simulink model "thermostat_model"  (R2024a)
settings: Solver=VariableStepAuto  StartTime=0.0  StopTime=10.0  RelTol=1e-3
StartFcn:
  | learning.simulink.modelCallbacks.startFunction(gcs)
StopFcn:
  | learning.simulink.modelCallbacks.stopFunction(gcs);
model workspace (MAT data in the model file):
  courseObject.course = 'simulink'
  courseObject.chapter = 12
  courseObject.lesson = 1
  courseObject.section = 3
  courseObject.task = 1
  t_ans = [0; 3.44882310802e-07; 2.06929386481e-06; 1.06913516349e-05; 5.38016404852e-05; 0.000269353084737; 0.00134711030599; 0.00673589641228; 0.0246147261548; 0.0493860964287; 0.083811385317; 0.129621810728; 0.15; 0.22645050849; 0.3; 0.398234685339; 0.45; 0.55; 0.6; 0.7; 0.75; 0.85; 0.9; 1; 1.05; 1.15; 1.2; 1.3; 1.35; 1.45; 1.5; 1.6; 1.65; 1.75; 1.8; 1.9; 1.95; 2.05; 2.1; 2.2; 2.25; 2.35; 2.4; 2.5; 2.55; 2.65; 2.7; 2.8; 2.85; 2.95; 3; 3.1; 3.15; 3.25; 3.3; 3.4; 3.45; 3.55; 3.6; 3.7; 3.75; 3.85; 3.9; 4; 4.05; 4.15; 4.2; 4.3; 4.35; 4.45; 4.5; 4.6; 4.65; 4.75; 4.8; 4.9; 4.95; 5.05; 5.1; 5.2; 5.25; 5.35; 5.4; 5.5; 5.55; 5.65; 5.7; 5.8; 5.85; 5.95; 6; 6.1; 6.15; 6.25; 6.3; 6.4; 6.45; 6.55; 6.6; 6.7; 6.75; 6.85; 6.9; 7; 7.05; 7.15; 7.2; 7.3; 7.35; 7.45; 7.5; 7.6; 7.65; 7.75; 7.8; 7.9; 7.95; 8.05; 8.1; 8.2; 8.25; 8.35; 8.4; 8.5; 8.55; 8.65; 8.7; 8.8; 8.85; 8.95; 9; 9.1; 9.15; 9.25; 9.3; 9.4; 9.45; 9.55; 9.6; 9.7; 9.75; 9.85; 9.9; 10]
  y_ans5 = [0.165; 0.164998492878; 0.164990957572; 0.164953288613; 0.164765132939; 0.163829066348; 0.159264513798; 0.139100169013; 0.2995349504; 0.280074861211; 0.411854808282; 0.399795884174; 0.507975423128; 0.592283569821; 0.667978066267; 0.737391490069; 0.802224756514; 0.863718172807; 0.922776170802; 0.980058262091; 1.03604536244; 1.09108815556; 1.14544235997; 1.19929444559; 1.25278038625; 1.30599933405; 1.35902359069; 1.41190587857; 1.46468464284; 1.51738791771; 1.57003614572; 1.62264423356; 1.6752230512; 1.72778052502; 1.78032243492; 1.83285299561; 1.88537528046; 1.93789153057; 1.99040338015; 2.04291202086; 2.09541832167; 2.14792291622; 2.20042626656; 2.25292870963; 2.30543049112; 2.35793179018; 2.41043273745; 2.4629334282; 2.5154339319; 2.56793429919; 2.62043456702; 2.67293476233; 2.72543490474; 2.77793500859; 2.83043508432; 2.88293513954; 2.9354351798; 2.98793520917; 3.04043523058; 3.09293524619]
  y_ans6 = [0; 0.000200949591965; 0.00120565787659; 0.00622820760954; 0.0313161877119; 0.156139821616; 0.765211136192; 3.47456129023; 9.66726186092; 14.4061638265; 17.7295717319; 19.7232109637; 20.7317148909; 20.8320685771; 21.5492269455; 21.892543187; 21.9704589902; 22.0381744411; 22.0479848156; 22.0487790728; 22.0492616288; 22.0494820492; 22.0494809578; 22.0492919817; 22.0489432093; 22.0484582994; 22.0478573326; 22.0471574743; 22.046373495; 22.045518183; 22.0446026738; 22.0436367161; 22.0426288871; 22.0415867683; 22.04051709; 22.0394258499; 22.0383184121; 22.0371995888; 22.0360737088; 22.0349446741; 22.0338160089; 22.0326908988; 22.0315722257; 22.030462596; 22.0293643652; 22.028279659; 22.0272103905; 22.0261582765; 22.0251248498; 22.024111472; 22.0231193432; 22.022149512; 22.0212028836; 22.0202802279; 22.0193821871; 22.0185092827; 22.0176619222; 22.0168404059; 22.0160449331; 22.0152756085; 22.0145324487; 22.0138153878; 22.0131242841; 22.0124589253; 22.0118190352; 22.0112042789]
  y_ans7 = [0 0.000200949591965 0.00120565787659 0.00622820760954 0.0313161877119 0.156139821616 0.765211136192 3.47456129023 9.66726186092 14.4061638265 17.7295717319 19.7232109637 ... (144 elements, 144x1)]
undefined symbols (not defined in the file): Ki, Kp, Ts
CloseFcn:
  | learning.simulink.cleanupOnlineTraining;learning.simulink.Application.getInstance().dduxLogMatlabEvent("ModelClosed")
Description:
  | TrainingCourseModel
settings Model: Creator=hp  LastModifiedBy=hp
settings DataIOCC: SaveTime=off
settings RTWCC: GPUComputeCapability=3.5

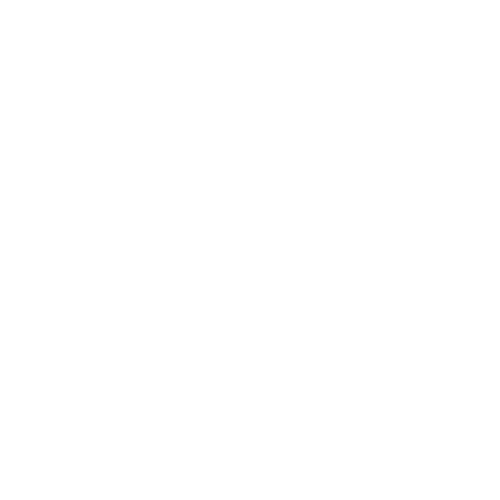
[thumbnail: Simulink's stored preview of the top-level diagram]
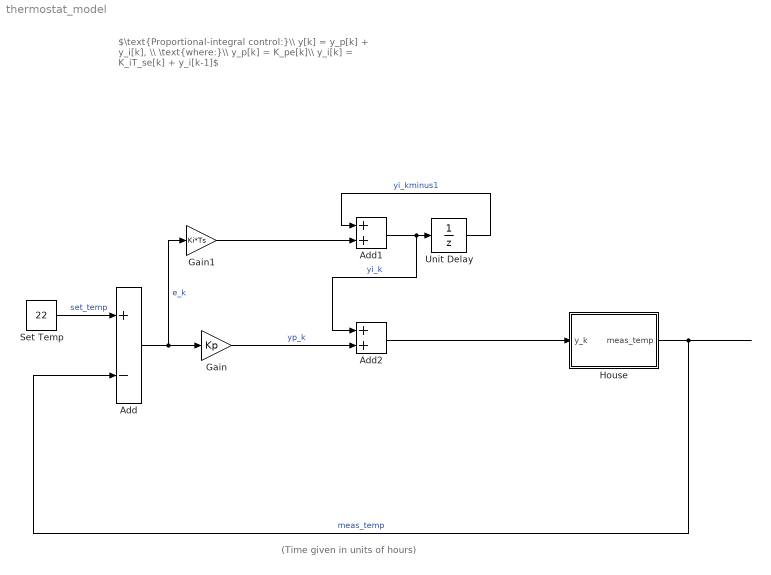
== system thermostat_model ==
  note: $\text{Proportional-integral control:}\\ y[k] = y_p[k] + y_i[k], \\ \text{where:}\\ y_p[k] = K_pe[k]\\ y_i[k] = K_iT_se[k] + y_i[k-1]$
  note: (Time given in units of hours)
  Add : Sum  Inputs=+-
  Add1 : Sum
  Add2 : Sum
  Gain : Gain  Gain=Kp
  Gain1 : Gain  Gain=Ki*Ts
  House : Subsystem
  Set Temp : Constant  Value=22
  Unit Delay : UnitDelay  SampleTime=Ts  HasFrameUpgradeWarning=on
  wires:
  House/1(meas_temp) -> Add/2  "meas_temp"
  Add/1 -> Gain1/1, Gain/1  "e_k"
  Set Temp/1 -> Add/1  "set_temp"
  Gain/1 -> Add2/2  "yp_k"
  Unit Delay/1 -> Add1/1  "yi_kminus1"
  Add1/1 -> Add2/1, Unit Delay/1  "yi_k"
  Gain1/1 -> Add1/2
  Add2/1 -> House/1(y_k)

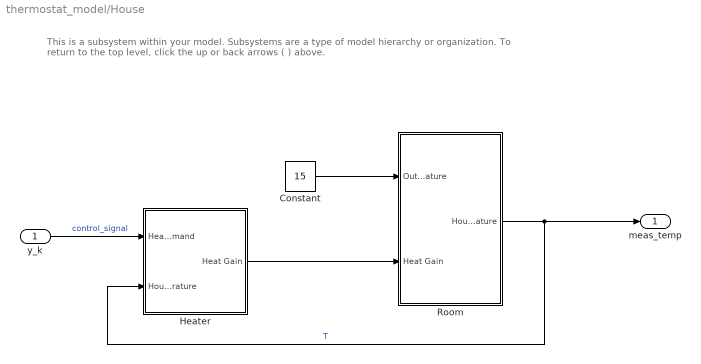
== system thermostat_model/House ==
  note: This is a subsystem within your model. Subsystems are a type of model hierarchy or organization.
      |
      | To return to the top level, click the up or back arrows ( ) above.
  y_k : Inport
  Constant : Constant  Value=15
  Heater : Subsystem
  Room : Subsystem
  meas_temp : Outport  VectorParamsAs1DForOutWhenUnconnected=off
  wires:
  y_k/1 -> Heater/1(Heater Command)  "control_signal"
  Heater/1(Heat Gain) -> Room/2("Heat Gain ")
  Room/1(House Temperature) -> meas_temp/1, Heater/2(House Temperature)  "T"
  Constant/1 -> Room/1(Outside Temperature)

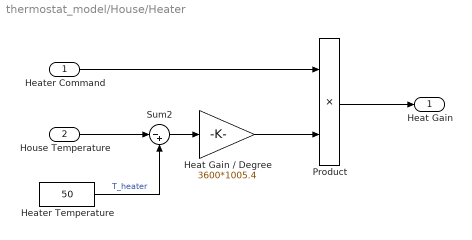
== system thermostat_model/House/Heater ==
  Heater Command : Inport
  House Temperature : Inport  Port=2
  Heat Gain / Degree : Gain  Gain=3600*1005.4
  Heater Temperature : Constant  Value=50
  Product : Product  RndMeth=Zero
  Sum2 : Sum  Inputs=|-+
  Heat Gain : Outport  Unit=joule/hour  VectorParamsAs1DForOutWhenUnconnected=off
  wires:
  Product/1 -> Heat Gain/1
  Heater Command/1 -> Product/1
  Heat Gain / Degree/1 -> Product/2
  Sum2/1 -> Heat Gain / Degree/1
  House Temperature/1 -> Sum2/1
  Heater Temperature/1 -> Sum2/2  "T_heater"

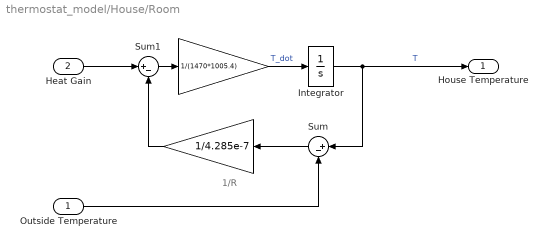
== system thermostat_model/House/Room ==
  note: 1/R
  Outside Temperature : Inport  Unit=°C
  "Heat Gain " : Inport  Port=2  Unit=joule/h
  " " : Gain  Gain=1/4.285e-7  SaturateOnIntegerOverflow=on  OutDataTypeStr=Inherit: Same as input  ParamDataTypeStr=Inherit: Same as input
  "  " : Gain  Gain=1/(1470*1005.4)  SaturateOnIntegerOverflow=on  OutDataTypeStr=Inherit: Same as input  ParamDataTypeStr=Inherit: Same as input
  Integrator : Integrator
  Sum : Sum  Inputs=|+-
  Sum1 : Sum  Inputs=|+-  InputSameDT=on  SaturateOnIntegerOverflow=on  OutDataTypeStr=Inherit: Same as first input
  House Temperature : Outport  Unit=°C  VectorParamsAs1DForOutWhenUnconnected=off
  wires:
  Outside Temperature/1 -> Sum/2
  Sum/1 -> " "/1
  " "/1 -> Sum1/2
  Integrator/1 -> House Temperature/1, Sum/1  "T"
  "  "/1 -> Integrator/1  "T_dot"
  Sum1/1 -> "  "/1
  "Heat Gain "/1 -> Sum1/1
